simulink model "invpend_NL_LQR"  (R2023b)
settings: Solver=VariableStepAuto  StartTime=0.0  StopTime=10.0  MaxStep=0.01  RelTol=1e-3
settings Model: Creator=bwang-ccny  LastModifiedBy=bwang-ccny

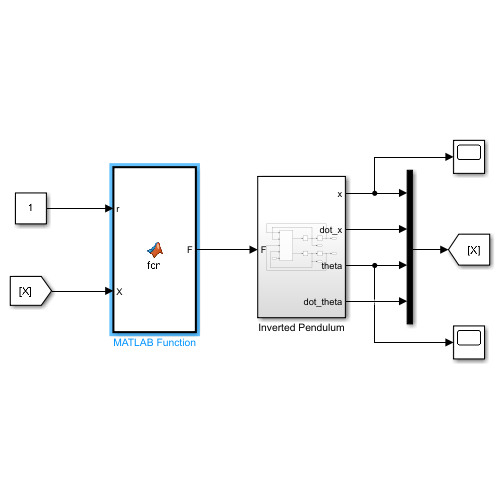
[thumbnail: Simulink's stored preview of the top-level diagram]
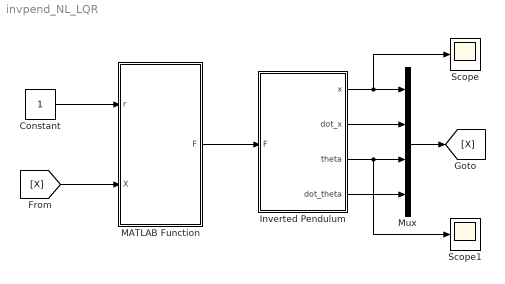
== system invpend_NL_LQR ==
  Constant : Constant
  Inverted Pendulum : Subsystem
  MATLAB Function : MATLAB Function  TreatAsAtomicUnit=on
  Mux : Mux
  Scope : Scope
  Scope1 : Scope
  wires:
  MATLAB Function/1(F) -> Inverted Pendulum/1(F)
  Constant/1 -> MATLAB Function/1(r)
  Inverted Pendulum/1(x) -> Scope/1, Mux/1
  Inverted Pendulum/2(dot_x) -> Mux/2
  Inverted Pendulum/3(theta) -> Scope1/1, Mux/3
  Inverted Pendulum/4(dot_theta) -> Mux/4
  Mux/1 -> [X]
  [X] -> MATLAB Function/2(X)

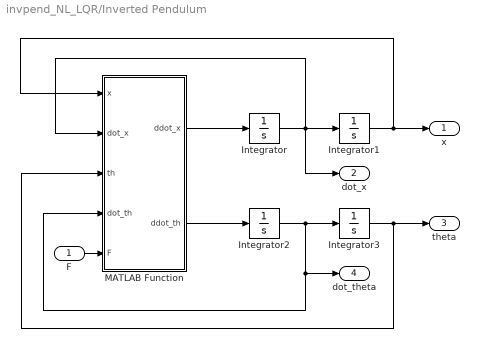
== system invpend_NL_LQR/Inverted Pendulum ==
  F : Inport
  Integrator{,1..3} (4 alike) : Integrator
  MATLAB Function : MATLAB Function  TreatAsAtomicUnit=on
  x : Outport
  dot_x : Outport  Port=2
  theta : Outport  Port=3
  dot_theta : Outport  Port=4
  wires:
  Integrator/1 -> dot_x/1, MATLAB Function/2(dot_x), Integrator1/1
  MATLAB Function/2(ddot_th) -> Integrator2/1
  Integrator2/1 -> dot_theta/1, MATLAB Function/4(dot_th), Integrator3/1
  Integrator1/1 -> x/1, MATLAB Function/1(x)
  Integrator3/1 -> theta/1, MATLAB Function/3(th)
  MATLAB Function/1(ddot_x) -> Integrator/1
  F/1 -> MATLAB Function/5(F)

== matlab function invpend_NL_LQR/MATLAB Function ==
  data: r input; F output; X input
function F = fcn(r, X)

x = X(1);
dot_x = X(2);
th = X(3);
dot_th = X(4);

%% LQR
K = [-1.0000   -1.5525  -18.6696   -3.4562];
F = -K*[(x - r), dot_x, th, dot_th]';

== matlab function invpend_NL_LQR/Inverted Pendulum/MATLAB Function ==
  data: x input; ddot_x output; dot_x input; th input; dot_th input; ddot_th output; F input
function [ddot_x, ddot_th] = fcn(x,dot_x,th,dot_th,F)

M = 0.5;
m = 0.2;
I = 0.006;
g = 9.8;
l = 0.3;
Q = (M + m)*(I + m*l^2) - (m*l)^2*cos(th)^2;


ddot_x = ((I + m*l^2)*(F + m*l*dot_th^2*sin(th)) - m^2*l^2*g*cos(th)*sin(th))/Q;
ddot_th = (m*l*cos(th)*F + m^2*l^2*dot_th^2*sin(th)*cos(th) - (M + m)*m*l*g*sin(th))/(-Q);
